simulink model "CoolingCheese_5thPoint"  (R2024a)
settings: Solver=VariableStepAuto  StartTime=0.0  StopTime=H  RelTol=1e-3
values from neighbouring files (symbols this model uses):
  C_f1 = c_f * m_f1    (= 1846687500)    [init.m]
  C_f2 = c_f * m_f2    (= 492450000)    [init.m]
  kaf1 = t_t * Sm1_ext    (= 4731)    [init.m]
  kaf2 = t_t * Sm2_ext    (= 1311)    [init.m]
  kaf_int = t_t * Sm_int    (= 171)    [init.m]
  qMAX_m1 = 25000    [init.m]
  qmin_m1 = -25000    [init.m]
  theta0_a = 291    [init.m]
  Ts = 1    [init.m]
  var_wf1 = 1    [init.m]
  var_wf2 = 1    [init.m]
libraries: slpidlib x1
settings Model: Creator=mrnel  LastModifiedBy=loren
settings ModelReferenceCC: EnableRefExpFcnMdlSchedulingChecks=on
settings RTWCC: GPUComputeCapability=3.5

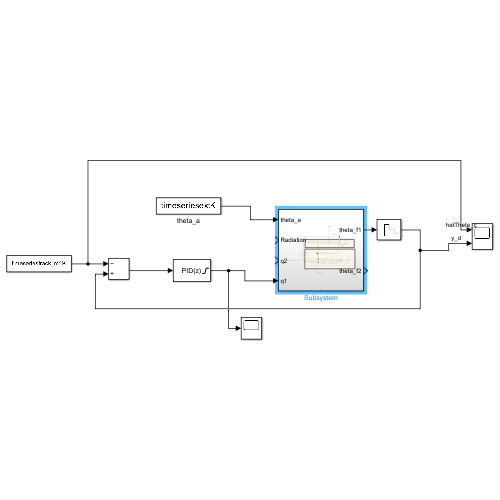
[thumbnail: Simulink's stored preview of the top-level diagram]
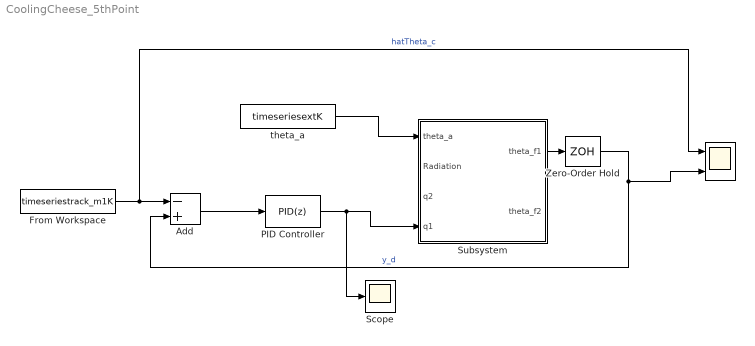
== system CoolingCheese_5thPoint ==
  " " : Scope  NumInputPorts=2
  Add : Sum  Inputs=-+
  From Workspace : FromWorkspace  VariableName=timeseriestrack_m1K  SampleTime=Ts
  PID Controller : slpidlib/PID Controller  Controller=PID  Form=Parallel  TimeDomain=Discrete-time  UseExternalTs=off  SampleTime=Ts  IntegratorMethod=Forward Euler  FilterMethod=Forward Euler  ControllerParametersSource=internal  P=-395607125.695296  I=-17119241.0275258  UseKiTs=off  D=-884178781.359412  UseExternalDerivativeSource=off  N=0.247171507358264  UseFilter=on  TunerSelectOption=Transfer Function Based (PID Tuner App)  InitialConditionSource=internal  InitialConditionForIntegrator=0  InitialConditionForFilter=0  DifferentiatorICPrevScaledInput=0  ExternalReset=none  TrackingMode=off  Kt=1  LimitOutput=on  SatLimitsSource=internal  UpperSaturationLimit=qMAX_m1  LowerSaturationLimit=qmin_m1  LinearizeAsGain=on  AntiWindupMode=none  Kb=1  LimitIntegrator=off  UpperIntegratorSaturationLimit=inf  LowerIntegratorSaturationLimit=-inf  POutMin=[]  POutMax=[]  IOutMin=[]  IOutMax=[]  DOutMin=[]  DOutMax=[]  NOutMin=[]  NOutMax=[]  SumOutMin=[]  SumOutMax=[]  SaturationOutMin=[]  SaturationOutMax=[]  PParamMin=[]  PParamMax=[]  IParamMin=[]  IParamMax=[]  DParamMin=[]  DParamMax=[]  NParamMin=[]  NParamMax=[]  KbParamMin=[]  KbParamMax=[]  KtParamMin=[]  KtParamMax=[]  KbOutMin=[]  KbOutMax=[]  KtOutMin=[]  KtOutMax=[]  IntegratorOutMin=[]  IntegratorOutMax=[]  FilterOutMin=[]  FilterOutMax=[]  SumI1OutMin=[]  SumI1OutMax=[]  SumI2OutMin=[]  SumI2OutMax=[]  SumI3OutMin=[]  SumI3OutMax=[]  SumI4OutMin=[]  SumI4OutMax=[]  SumDOutMin=[]  SumDOutMax=[]  DifferentiatorOutMin=[]  DifferentiatorOutMax=[]  FilterDiffOutCoefMin=[]  FilterDiffOutCoefMax=[]  ReciprocalOutMin=[]  ReciprocalOutMax=[]  SumDenOutMin=[]  SumDenOutMax=[]  SumNumOutMin=[]  SumNumOutMax=[]  DivideOutMin=[]  DivideOutMax=[]  UdiffTsProdOutMin=[]  UdiffTsProdOutMax=[]  NTsProdOutMin=[]  NTsProdOutMax=[]  UintegralTsProdOutMin=[]  UintegralTsProdOutMax=[]  UngainTsProdOutMin=[]  UngainTsProdOutMax=[]  ClampingZeroOutDataTypeStr=Inherit: Inherit via back propagation  ClampingZeroOutMin=[]  ClampingZeroOutMax=[]  FilterDenConstantOutDataTypeStr=Inherit: Inherit via back propagation  FilterDenConstantOutMin=[]  FilterDenConstantOutMax=[]  PCopyOutDataTypeStr=Inherit: Inherit via back propagation  PCopyOutMin=[]  PCopyOutMax=[]  NCopyOutDataTypeStr=Inherit: Inherit via back propagation  NCopyOutMin=[]  NCopyOutMax=[]  IntegratorContinuousStateAttributes=''  IntegratorStateMustResolveToSignalObject=off  IntegratorRTWStateStorageClass=Auto  FilterContinuousStateAttributes=''  FilterStateMustResolveToSignalObject=off  FilterRTWStateStorageClass=Auto  ParallelPVariant=InternalParameters  IdealPVariant=Disabled  IVariant=InternalParameters  DVariant=InternalParameters  IntegratorVariant=Discrete  SatVariant=Enabled  AWVariant=Passthrough  PCopyVariant=Disabled  TRVariant=Disabled  FdbkBlocksVariant=Forward  IdealPFdbkVariant=Disabled  SatFdbkVariant=Disabled  DerivativeFilterVariant=ForwardEulerFilter  NVariant=InternalParameters  NCopyVariant=Disabled  FilterICVariant=InternalICsFilter  IntegratorICVariant=InternalICs  ExternalResetVariant=Disabled  TRSumVariant=Passthrough  SumFdbkVariant=Disabled  SumVariant=Sum_PID  TsampFilterVariant=InternalTs  TsampNgainVariant=Passthrough  TsampIntegralVariant=Disabled_SignalSpec  ExternalSaturationOutDataTypeStr=Inherit: Same as second input  DerivativeSourceVariant=ErrorSignal
  Scope : Scope
  Subsystem : Subsystem
  Zero-Order Hold : ZeroOrderHold  SampleTime=Ts
  theta_a : FromWorkspace  VariableName=timeseriesextK  SampleTime=Ts
  wires:
  theta_a/1 -> Subsystem/1(theta_a)
  PID Controller/1 -> Scope/1, Subsystem/4(q1)
  Subsystem/1(theta_f1) -> Zero-Order Hold/1
  Zero-Order Hold/1 -> Add/2, " "/2  "y_d"
  From Workspace/1 -> " "/1, Add/1  "hatTheta_c"
  Add/1 -> PID Controller/1

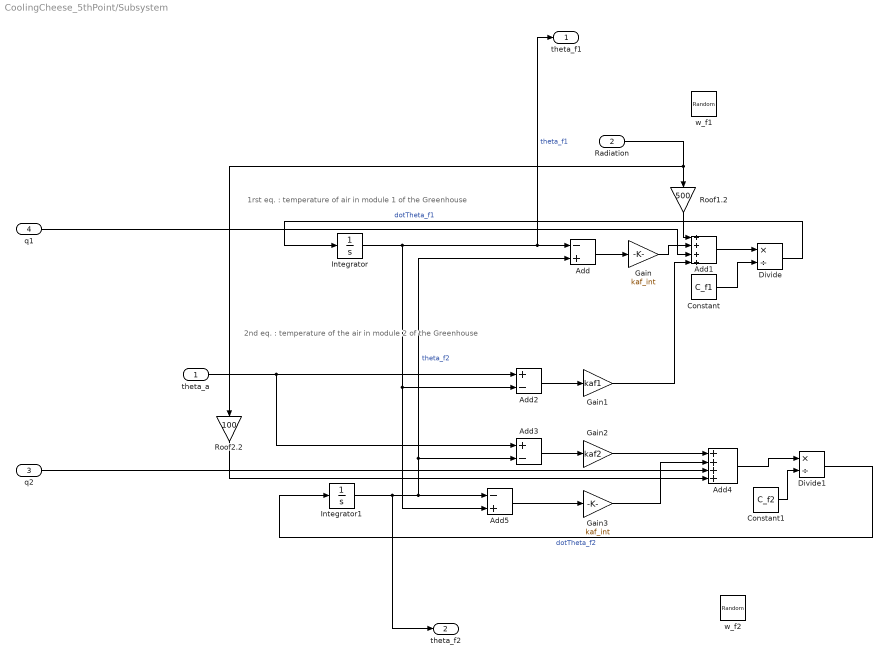
== system CoolingCheese_5thPoint/Subsystem ==
  note: 1rst eq. : temperature of air in module 1 of the Greenhouse
  note: 2nd eq. : temperature of the air in module 2 of the Greenhouse
  theta_a : Inport
  Radiation : Inport  Port=2
  q2 : Inport  Port=3
  q1 : Inport  Port=4
  Add : Sum  Inputs=-+
  Add1 : Sum  Inputs=++++
  Add2 : Sum  Inputs=+-
  Add3 : Sum  Inputs=+-
  Add4 : Sum  Inputs=++++
  Add5 : Sum  Inputs=-+
  Constant : Constant  Value=C_f1
  Constant1 : Constant  Value=C_f2
  Divide : Product  Inputs=*/
  Divide1 : Product  Inputs=*/
  Gain : Gain  Gain=kaf_int
  Gain1 : Gain  Gain=kaf1
  Gain2 : Gain  Gain=kaf2
  Gain3 : Gain  Gain=kaf_int
  Integrator : Integrator  InitialCondition=theta0_a
  Integrator1 : Integrator  InitialCondition=theta0_a
  Roof1.2 : Gain  Gain=500
  Roof2.2 : Gain  Gain=100
  w_f1 : RandomNumber  Variance=var_wf1  SampleTime=Ts
  w_f2 : RandomNumber  Variance=var_wf2  SampleTime=Ts
  theta_f1 : Outport
  theta_f2 : Outport  Port=2
  wires:
  Add1/1 -> Divide/1
  Add3/1 -> Gain2/1
  Divide1/1 -> Integrator1/1  "dotTheta_f2"
  Roof1.2/1 -> Add1/1
  Gain/1 -> Add1/2
  Integrator1/1 -> theta_f2/1, Add3/2, Add/2, Add5/1  "theta_f2"
  Gain1/1 -> Add1/4
  Constant/1 -> Divide/2
  Gain3/1 -> Add4/2
  Constant1/1 -> Divide1/2
  Divide/1 -> Integrator/1  "dotTheta_f1"
  Radiation/1 -> Roof2.2/1, Roof1.2/1
  Add4/1 -> Divide1/1
  Add2/1 -> Gain1/1
  Add/1 -> Gain/1
  Gain2/1 -> Add4/1
  Add5/1 -> Gain3/1
  Roof2.2/1 -> Add4/4
  q1/1 -> Add1/3
  theta_a/1 -> Add3/1, Add2/1
  Integrator/1 -> Add5/2, Add2/2, theta_f1/1, Add/1  "theta_f1"
  q2/1 -> Add4/3
